simulink model "GFL_test"  (R2019b)
settings: Solver=ode1  StartTime=0.0  StopTime=10.0  FixedStep=Ts  MaxStep=1e-4  RelTol=1e-3
undefined symbols (not defined in the file): Ts
libraries: powerlib x5, GFe_Lib x1, VSC_Lib x1
settings Model: Creator=Frederic_Colas  LastModifiedBy=Frederic_Colas
settings DataIOCC: ReturnWorkspaceOutputs=off
settings DebuggingCC: UnconnectedInputMsg=none  UnconnectedOutputMsg=none  UnconnectedLineMsg=none  ArithmeticOperatorsInVariantConditions=warning
settings SFSimCC: SimUseLocalCustomCode=off  CustomCodeUndefinedFunction=UseInterfaceOnly
settings RTWCC: RTWUseLocalCustomCode=off

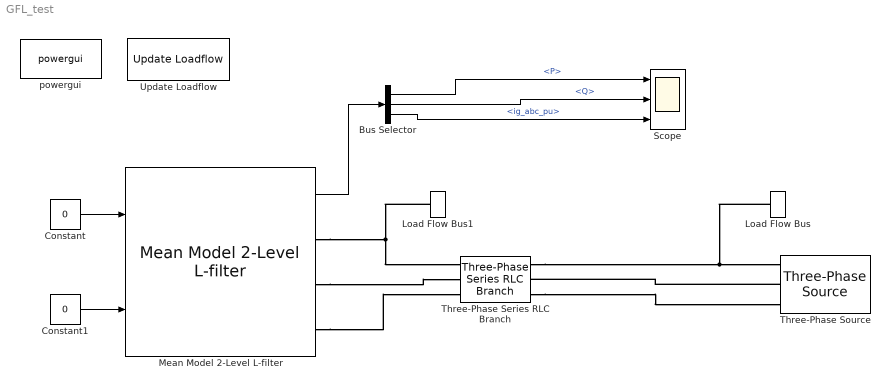
== system GFL_test ==
  Bus Selector : BusSelector  OutputSignals=P,Q,I.ig_abc_pu
  Constant : Constant  Value=0
  Constant1 : Constant  Value=0
  Load Flow Bus : powerlib/Measurements/Load Flow Bus  LConnTagsString=a  Phases=single  Connectors=on one side  ID=BUS_1  Vbase=400  Vref=1  Vangle=0  VLF=1  VLFb=1  VLFc=1  angleLF=0  angleLFb=0  angleLFc=0
  Load Flow Bus1 : powerlib/Measurements/Load Flow Bus  LConnTagsString=a  Phases=single  Connectors=on one side  ID=BUS_2  Vbase=400  Vref=1  Vangle=0  VLF=1.001  VLFb=1  VLFc=1  angleLF=0.2249  angleLFb=0  angleLFc=0
  Mean Model 2-Level L-filter : GFe_Lib/Mean Model 2-Level L-filter  fn=50  Sn=10e3  Pn=10e3  Udcn=750  Time_Step=Ts  Un1=400  Un2=400  m=1  Rt_pu=0.005  Lt_pu=0.15  Lm_pu=500  Rm_pu=500  Tr_PLL=10  wn_i=1500  zeta_i=1  Kffi=on  Filtre_FF=on  w_ff=1000  QV=Reactive Power Control  w_P=10  w_V=50  w_LPF=4000  Imax=5  Iqmax=5  K_FRT=0  LFpopup=PQ  P0=0.2  Q0=0  V0=1.0006  Theta0=0.22486
      settings: SourceProductName=VSC4SPS
  Scope : Scope  NumInputPorts=3
  Three-Phase Series RLC Branch : powerlib/Elements/Three-Phase Series RLC Branch  LConnTagsString=A|B|C  RConnTagsString=A|B|C  BranchType=RL  Resistance=0.05  Inductance=1e-3  Capacitance=1e-6  Measurements=None
  Three-Phase Source : powerlib/Electrical Sources/Three-Phase Source  InternalConnection=Yg  VoltagePhases=off  Voltage=(400)*1  PhaseAngle=0  Voltage_phases=[25e3 25e3 25e3]/sqrt(3)  PhaseAngles_phases=[0 -120 +120]  Frequency=50  NonIdealSource=off  SpecifyImpedance=off  Resistance=0.8929  Inductance=16.58e-3  ShortCircuitLevel=100e6  BaseVoltage=25e3  XRratio=7  BusType=swing  Pref=10e3  Qref=0  Prefabc=[10e3, 10e3, 10e3]  Qrefabc=[0, 0, 0]  Qmin=-inf  Qmax=inf
  Update Loadflow : VSC_Lib/Update Loadflow  ShowInLibBrowser=on
      settings: SourceProductName=VSC4SPS
  powergui : powerlib/powergui  Priority=1  SimulationMode=Discrete  SampleTime=Ts  frequency=60  Iterations=50  frequencyindice=50  Pbase=10000  ErrMax=1e-6  UnitsV=kV  UnitsW=kW  buscounter=0  FunctionMessages=off  echomessages=off  EnableUseOfTLC=off  CurrentSourceSwitches=off  DisableSnubberDevices=off  DisableRonSwitches=off  DisableVfSwitches=off  DisplayEquations=off  AutomaticDiscreteSolvers=off  SolverType=Tustin/Backward Euler (TBE)  Interpol=off  ExternalGateDelay=off  methode=off  Ts=100  x0status=blocks  SPID=on  SwTol=0  HookPort=off  NonlinearTolerance=1e-4  nMaxIteration=100  ContinueOnMaxIteration=off  RestoreLinks=warning  ResistiveCurrentMeasurement=off  Frange=[0:2:500]  Ylog=off  Xlog=on  ShowGrid=off  save=off  variable=ZData  structure=0  ZoomFFT=off  StartTime=0.0  cycles=1  DisplayStyle=1  fundamental=60  FreqAxis=off  MaxFrequency=1000  frequencyindicesteady=1  RmsSteady=1  display=off
  wires:
  Mean Model 2-Level L-filter/1 -> Bus Selector/1
  Bus Selector/1 -> Scope/1  "<P>"
  Bus Selector/2 -> Scope/2  "<Q>"
  Bus Selector/3 -> Scope/3  "<ig_abc_pu>"
  Constant/1 -> Mean Model 2-Level L-filter/1
  Constant1/1 -> Mean Model 2-Level L-filter/2
  connections:
  Mean Model 2-Level L-filter/RConn1 -- Three-Phase Series RLC Branch/LConn1 -- Load Flow Bus1/LConn1
  Mean Model 2-Level L-filter/RConn2 -- Three-Phase Series RLC Branch/LConn2
  Mean Model 2-Level L-filter/RConn3 -- Three-Phase Series RLC Branch/LConn3
  Three-Phase Series RLC Branch/RConn1 -- Load Flow Bus/LConn1 -- Three-Phase Source/RConn1
  Three-Phase Source/RConn2 -- Three-Phase Series RLC Branch/RConn2
  Three-Phase Series RLC Branch/RConn3 -- Three-Phase Source/RConn3
